simulink model "variable_estado_continuo"  (R2015a)
settings: Solver=ode45  StartTime=0.0  StopTime=20  RelTol=1e-3
values from neighbouring files (symbols this model uses):
  A = double(subs(A,[R L Kv Kf m1 k1 b1 m2 m3 b2 b3 k2],ones(1,12)))    [primerparcial.m]
  Ad = sysd(1,1).a    [primerparcial.m]
  B = double(subs(B,[R L Kv Kf m1 k1 b1 m2 m3 b2 b3 k2],ones(1,12)))    [primerparcial.m]
  Bd = [sysd(1,1).b sysd(1,2).b]    [primerparcial.m]
  C = double(C)    [primerparcial.m]
  Cd = [sysd(1,1).c ;sysd(2,1).c]    [primerparcial.m]
  Ts = 1/(pc*10)    [primerparcial.m]
settings Model: CovSFcnEnable=off  Creator=Jose  LastModifiedBy=carma_000
settings DebuggingCC: SolverPrmCheckMsg=warning

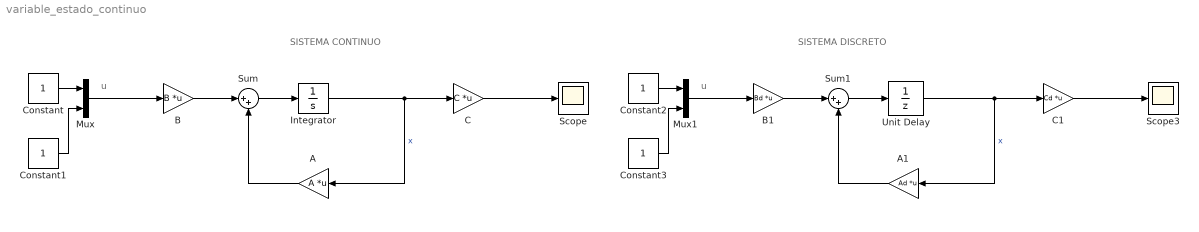
== system variable_estado_continuo ==
  note: SISTEMA CONTINUO
  note: u
  note: u
  note: SISTEMA DISCRETO
  A : Gain  Gain=A  Multiplication=Matrix(K*u)
  A1 : Gain  Gain=Ad  Multiplication=Matrix(K*u)  SampleTime=Ts
  B : Gain  Gain=B  Multiplication=Matrix(K*u)
  B1 : Gain  Gain=Bd  Multiplication=Matrix(K*u)  SampleTime=Ts
  C : Gain  Gain=C  Multiplication=Matrix(K*u)
  C1 : Gain  Gain=Cd  Multiplication=Matrix(K*u)  SampleTime=Ts
  Constant : Constant
  Constant1 : Constant
  Constant2 : Constant  SampleTime=Ts
  Constant3 : Constant  SampleTime=Ts
  Integrator : Integrator
  Mux : Mux  Inputs=2
  Mux1 : Mux  Inputs=2
  Scope : Scope
      settings: ShowLegends=on  TimeRange=10
  Scope3 : Scope
      settings: ShowLegends=on  TimeRange=10  SaveName=ScopeData3
  Sum : Sum  Inputs=|++
  Sum1 : Sum  Inputs=|++
  Unit Delay : UnitDelay  SampleTime=Ts
  wires:
  B/1 -> Sum/1
  Sum/1 -> Integrator/1
  Integrator/1 -> C/1, A/1  "x"
  A/1 -> Sum/2
  C/1 -> Scope/1
  Constant1/1 -> Mux/2
  Constant/1 -> Mux/1
  Mux/1 -> B/1
  B1/1 -> Sum1/1
  Sum1/1 -> Unit Delay/1
  Unit Delay/1 -> C1/1, A1/1  "x"
  A1/1 -> Sum1/2
  C1/1 -> Scope3/1
  Constant3/1 -> Mux1/2
  Constant2/1 -> Mux1/1
  Mux1/1 -> B1/1
